simulink model "moto_linearization"  (R2026a)
settings: Solver=VariableStepAuto  StopTime=30
values from neighbouring files (symbols this model uses):
  ft = bs.FrontTire    [bikeSimToMotoParameters.m]
  Gf = Nsh.'*(Oh - B)    [bikeSimToMotoParameters.m]
  Ib = sum(I,3)    [bikeSimToMotoParameters.m]
  If = sum(I,3)    [bikeSimToMotoParameters.m]
  Ift = zeros(3)    [bikeSimToMotoParameters.m]
  Irt = zeros(3)    [bikeSimToMotoParameters.m]
  m = front_bodies(k).m    [bikeSimToMotoParameters.m]
  N = eye(3)    [bikeSimToMotoParameters.m]
  Ob = sum([rear_bodies.O].*[rear_bodies.m],2)/p.mb    [bikeSimToMotoParameters.m]
  p = motoParameters    [bikeSimToMotoParameters.m]    (also in moto_init.m = bikeSimToPrydeV2Parameters(bs,130/3.6); moto_trim_test.m = P{idx_vx}; steadyTurningTrimEqns.m = in3(41,:); steadyTurningTrimJac.m = in3(41,:))
  pf = fpacejka(bs.FrontTire.Pacejka)    [moto_trim_test.m]
  pr = fpacejka(bs.RearTire.Pacejka)    [moto_trim_test.m]
  rt = bs.RearTire    [bikeSimToMotoParameters.m]
  s = linspace(-pi,pi,36)'    [moto_init.m]
  sm = bs.SprungMass    [bikeSimToMotoParameters.m]
  X = zeros(ns,ns,12)    [moto_trim_test.m]
undefined symbols (not defined in the file or in its folder): mb, mh, Rr, Vlow, Y, Z
libraries: sm_lib x60, nesl_utility x51
(part 5 of 5)

== system moto_linearization/moto/Subsystem/front_tire/Subsystem1/Lateral force (pure slip)/Magic formula (lateral, camber) ==
  Bg : Inport
  Cg : Inport  Port=2
  Eg : Inport  Port=3
  camber : Inport  Port=4
  Atan : Trigonometry  Operator=atan
  Atan1 : Trigonometry  Operator=atan
  Product : Product
  Product1 : Product
  Product2 : Product
  Sum : Sum  Inputs=|+-
  Sum1 : Sum  Inputs=|+-
  Fy0g : Outport
  wires:
  Product2/1 -> Fy0g/1
  Eg/1 -> Product1/1
  Cg/1 -> Product2/1
  camber/1 -> Product/2
  Sum1/1 -> Atan1/1
  Product1/1 -> Sum1/2
  Sum/1 -> Product1/2
  Product/1 -> Sum1/1, Sum/1, Atan/1
  Atan1/1 -> Product2/2
  Atan/1 -> Sum/2
  Bg/1 -> Product/1

== system moto_linearization/moto/Subsystem/front_tire/Subsystem1/Lateral force (pure slip)/Magic formula (lateral, slip) ==
  By : Inport
  Cy : Inport  Port=2
  Ey : Inport  Port=3
  slip : Inport  Port=4
  Atan : Trigonometry  Operator=atan
  Atan1 : Trigonometry  Operator=atan
  Product : Product
  Product1 : Product
  Product2 : Product
  Sum : Sum  Inputs=|+-
  Sum1 : Sum  Inputs=|+-
  Fy0a : Outport
  wires:
  Product1/1 -> Sum1/2
  Sum1/1 -> Atan1/1
  slip/1 -> Product/2
  Atan/1 -> Sum/2
  Ey/1 -> Product1/1
  Atan1/1 -> Product2/2
  Product/1 -> Sum1/1, Sum/1, Atan/1
  Product2/1 -> Fy0a/1
  By/1 -> Product/1
  Sum/1 -> Product1/2
  Cy/1 -> Product2/1

== system moto_linearization/moto/Subsystem/front_tire/Subsystem1/Lateral force (pure slip)/lateral stiffness factor (camber, normalized) ==
  Kyg : Inport
  Cg : Inport  Port=2
  Dy : Inport  Port=3
  Divide : Product  Inputs=*/
  Product : Product
  Bg : Outport
  wires:
  Dy/1 -> Product/2
  Product/1 -> Divide/2
  Divide/1 -> Bg/1
  Cg/1 -> Product/1
  Kyg/1 -> Divide/1

== system moto_linearization/moto/Subsystem/front_tire/Subsystem1/Lateral force (pure slip)/lateral stiffness factor (slip, normalized) ==
  Kya : Inport
  Cy : Inport  Port=2
  Dy : Inport  Port=3
  Divide : Product  Inputs=*/
  Product : Product
  By : Outport
  wires:
  Cy/1 -> Product/1
  Dy/1 -> Product/2
  Kya/1 -> Divide/1
  Product/1 -> Divide/2
  Divide/1 -> By/1

== system moto_linearization/moto/Subsystem/front_tire/Subsystem1/Lateral force (pure slip, no camber)/Lateral curvature factor ==
  slip : Inport
  camber : Inport  Port=2
  pey1 : Inport  Port=3
  pey2 : Inport  Port=4
  pey4 : Inport  Port=5
  Product : Product  Inputs=3
  Product1 : Product
  Sign : Signum
  Square : Math  Operator=square
  Sum : Sum  Inputs=|++
  Sum1 : Sum  Inputs=|++
  Ey : Outport
  wires:
  slip/1 -> Sign/1
  pey1/1 -> Sum/1
  Sign/1 -> Product/1
  camber/1 -> Square/1, Product/3
  pey4/1 -> Product/2
  Product/1 -> Sum/2
  Sum/1 -> Sum1/1
  Square/1 -> Product1/1
  pey2/1 -> Product1/2
  Product1/1 -> Sum1/2
  Sum1/1 -> Ey/1

== system moto_linearization/moto/Subsystem/front_tire/Subsystem1/Lateral force (pure slip, no camber)/Lateral peak factor ==
  dfz : Inport
  Fz : Inport  Port=2
  camber : Inport  Port=3
  pdy1 : Inport  Port=4
  pdy2 : Inport  Port=5
  pdy3 : Inport  Port=6
  Constant : Constant
  Divide : Product  Inputs=*/
  Exp : Math
  Product : Product  Inputs=3
  Product1 : Product
  Product2 : Product
  Square : Math  Operator=square
  Sum : Sum  Inputs=|++
  Dy : Outport
  wires:
  Fz/1 -> Product/1
  pdy1/1 -> Product/2
  pdy2/1 -> Product1/1
  dfz/1 -> Product1/2
  Product1/1 -> Exp/1
  Exp/1 -> Product/3
  camber/1 -> Square/1
  pdy3/1 -> Product2/2
  Square/1 -> Product2/1
  Product/1 -> Divide/1
  Divide/1 -> Dy/1
  Product2/1 -> Sum/1
  Sum/1 -> Divide/2
  Constant/1 -> Sum/2

== system moto_linearization/moto/Subsystem/front_tire/Subsystem1/Lateral force (pure slip, no camber)/Lateral stiffness factor (camber) ==
  dfz : Inport
  Fz : Inport  Port=2
  pky6 : Inport  Port=3
  pky7 : Inport  Port=4
  Product : Product
  Product1 : Product
  Sum : Sum  Inputs=|++
  Kyg : Outport
  wires:
  pky7/1 -> Product/1
  dfz/1 -> Product/2
  Product/1 -> Sum/2
  pky6/1 -> Sum/1
  Sum/1 -> Product1/1
  Fz/1 -> Product1/2
  Product1/1 -> Kyg/1

== system moto_linearization/moto/Subsystem/front_tire/Subsystem1/Lateral force (pure slip, no camber)/Lateral stiffness factor (slip) ==
  Fz : Inport
  camber : Inport  Port=2
  Fz0 : Inport  Port=3
  pky1 : Inport  Port=4
  pky2 : Inport  Port=5
  pky3 : Inport  Port=6
  pky4 : Inport  Port=7
  pky5 : Inport  Port=8
  Atan : Trigonometry  Operator=atan
  Constant : Constant
  Divide : Product  Inputs=*/
  Divide1 : Product  Inputs=*/
  Product{,1..2,4} (4 alike) : Product
  Product3 : Product  Inputs=3
  Sin : Trigonometry
  Square : Math  Operator=square
  Sum : Sum  Inputs=|++
  Sum1 : Sum  Inputs=|++
  Kya : Outport
  wires:
  camber/1 -> Square/1
  Square/1 -> Product4/1, Product/2
  pky4/1 -> Product/1
  pky3/1 -> Sum/1
  Product/1 -> Sum/2
  Sum/1 -> Product1/2
  Fz0/1 -> Product3/2, Product1/1
  Product1/1 -> Divide/2
  Fz/1 -> Divide/1
  Divide/1 -> Atan/1
  Atan/1 -> Product2/2
  pky2/1 -> Product2/1
  Product2/1 -> Sin/1
  Sin/1 -> Product3/3
  pky1/1 -> Product3/1
  Product3/1 -> Divide1/1
  pky5/1 -> Product4/2
  Product4/1 -> Sum1/1
  Constant/1 -> Sum1/2
  Sum1/1 -> Divide1/2
  Divide1/1 -> Kya/1

== system moto_linearization/moto/Subsystem/front_tire/Subsystem1/Lateral force (pure slip, no camber)/Magic formula (lateral) ==
  Dy : Inport
  Fy0a : Inport  Port=2
  Fy0g : Inport  Port=3
  Product : Product
  Sin : Trigonometry
  Sum : Sum  Inputs=|++
  Fy0 : Outport
  wires:
  Fy0a/1 -> Sum/1
  Fy0g/1 -> Sum/2
  Sum/1 -> Sin/1
  Dy/1 -> Product/1
  Sin/1 -> Product/2
  Product/1 -> Fy0/1

== system moto_linearization/moto/Subsystem/front_tire/Subsystem1/Lateral force (pure slip, no camber)/Magic formula (lateral, camber) ==
  Bg : Inport
  Cg : Inport  Port=2
  Eg : Inport  Port=3
  camber : Inport  Port=4
  Atan : Trigonometry  Operator=atan
  Atan1 : Trigonometry  Operator=atan
  Product : Product
  Product1 : Product
  Product2 : Product
  Sum : Sum  Inputs=|+-
  Sum1 : Sum  Inputs=|+-
  Fy0g : Outport
  wires:
  Product2/1 -> Fy0g/1
  Eg/1 -> Product1/1
  Cg/1 -> Product2/1
  camber/1 -> Product/2
  Sum1/1 -> Atan1/1
  Product1/1 -> Sum1/2
  Sum/1 -> Product1/2
  Product/1 -> Sum1/1, Sum/1, Atan/1
  Atan1/1 -> Product2/2
  Atan/1 -> Sum/2
  Bg/1 -> Product/1

== system moto_linearization/moto/Subsystem/front_tire/Subsystem1/Lateral force (pure slip, no camber)/Magic formula (lateral, slip) ==
  By : Inport
  Cy : Inport  Port=2
  Ey : Inport  Port=3
  slip : Inport  Port=4
  Atan : Trigonometry  Operator=atan
  Atan1 : Trigonometry  Operator=atan
  Product : Product
  Product1 : Product
  Product2 : Product
  Sum : Sum  Inputs=|+-
  Sum1 : Sum  Inputs=|+-
  Fy0a : Outport
  wires:
  Product1/1 -> Sum1/2
  Sum1/1 -> Atan1/1
  slip/1 -> Product/2
  Atan/1 -> Sum/2
  Ey/1 -> Product1/1
  Atan1/1 -> Product2/2
  Product/1 -> Sum1/1, Sum/1, Atan/1
  Product2/1 -> Fy0a/1
  By/1 -> Product/1
  Sum/1 -> Product1/2
  Cy/1 -> Product2/1

== system moto_linearization/moto/Subsystem/front_tire/Subsystem1/Lateral force (pure slip, no camber)/lateral stiffness factor (camber, normalized) ==
  Kyg : Inport
  Cg : Inport  Port=2
  Dy : Inport  Port=3
  Divide : Product  Inputs=*/
  Product : Product
  Bg : Outport
  wires:
  Dy/1 -> Product/2
  Product/1 -> Divide/2
  Divide/1 -> Bg/1
  Cg/1 -> Product/1
  Kyg/1 -> Divide/1

== system moto_linearization/moto/Subsystem/front_tire/Subsystem1/Lateral force (pure slip, no camber)/lateral stiffness factor (slip, normalized) ==
  Kya : Inport
  Cy : Inport  Port=2
  Dy : Inport  Port=3
  Divide : Product  Inputs=*/
  Product : Product
  By : Outport
  wires:
  Cy/1 -> Product/1
  Dy/1 -> Product/2
  Kya/1 -> Divide/1
  Product/1 -> Divide/2
  Divide/1 -> By/1

== system moto_linearization/moto/Subsystem/front_tire/Subsystem1/Longitudinal force (combined slip)/Combined slip ==
  Bxa : Inport
  Cxa : Inport  Port=2
  Fx0 : Inport  Port=3
  slip_angle : Inport  Port=4
  Atan : Trigonometry  Operator=atan
  Cos : Trigonometry  Operator=cos
  Product : Product
  Product1 : Product
  Product2 : Product
  Fx : Outport
  wires:
  Bxa/1 -> Product/1
  slip_angle/1 -> Product/2
  Product/1 -> Atan/1
  Atan/1 -> Product1/1
  Cxa/1 -> Product1/2
  Product1/1 -> Cos/1
  Cos/1 -> Product2/1
  Fx0/1 -> Product2/2
  Product2/1 -> Fx/1

== system moto_linearization/moto/Subsystem/front_tire/Subsystem1/Longitudinal force (combined slip)/Longitudinal stiffness factor (combined) ==
  slip_ratio : Inport
  rbx1 : Inport  Port=2
  rbx2 : Inport  Port=3
  Atan : Trigonometry  Operator=atan
  Cos : Trigonometry  Operator=cos
  Product : Product
  Product1 : Product
  Bxa : Outport
  wires:
  slip_ratio/1 -> Product/1
  rbx2/1 -> Product/2
  Product/1 -> Atan/1
  Atan/1 -> Cos/1
  Cos/1 -> Product1/2
  rbx1/1 -> Product1/1
  Product1/1 -> Bxa/1

== system moto_linearization/moto/Subsystem/front_tire/Subsystem1/Longitudinal force (pure slip)/Longitudinal curvature factor ==
  dfz : Inport
  slip_ratio : Inport  Port=2
  pex1 : Inport  Port=3
  pex2 : Inport  Port=4
  pex3 : Inport  Port=5
  Constant : Constant
  Product : Product
  Product1 : Product
  Product2 : Product
  Sign : Signum
  Square : Math  Operator=square
  Sum : Sum  Inputs=|++
  Sum1 : Sum  Inputs=|++
  Sum2 : Sum  Inputs=|+-
  Ex : Outport
  wires:
  pex1/1 -> Sum/1
  Product/1 -> Sum/2
  pex2/1 -> Product/1
  dfz/1 -> Square/1, Product/2
  Square/1 -> Product1/1
  pex3/1 -> Product1/2
  Sum/1 -> Sum1/1
  Product1/1 -> Sum1/2
  Sum1/1 -> Product2/1
  Constant/1 -> Sum2/1
  Sum2/1 -> Product2/2
  Product2/1 -> Ex/1
  slip_ratio/1 -> Sign/1
  Sign/1 -> Sum2/2

== system moto_linearization/moto/Subsystem/front_tire/Subsystem1/Longitudinal force (pure slip)/Longitudinal peak factor ==
  dfz : Inport
  Fz : Inport  Port=2
  pdx1 : Inport  Port=3
  pdx2 : Inport  Port=4
  Product : Product
  Product1 : Product
  Sum : Sum  Inputs=|++
  Dx : Outport
  wires:
  dfz/1 -> Product/1
  pdx2/1 -> Product/2
  pdx1/1 -> Sum/1
  Product/1 -> Sum/2
  Fz/1 -> Product1/1
  Sum/1 -> Product1/2
  Product1/1 -> Dx/1

== system moto_linearization/moto/Subsystem/front_tire/Subsystem1/Longitudinal force (pure slip)/Longitudinal stiffness factor ==
  dfz : Inport
  Fz : Inport  Port=2
  pkx1 : Inport  Port=3
  pkx2 : Inport  Port=4
  pkx3 : Inport  Port=5
  Exp : Math
  Product : Product
  Product1 : Product
  Product2 : Product  Inputs=3
  Sum : Sum  Inputs=|++
  Kx : Outport
  wires:
  pkx2/1 -> Product/1
  dfz/1 -> Product1/1, Product/2
  pkx1/1 -> Sum/1
  Product/1 -> Sum/2
  pkx3/1 -> Product1/2
  Product1/1 -> Exp/1
  Fz/1 -> Product2/1
  Sum/1 -> Product2/2
  Exp/1 -> Product2/3
  Product2/1 -> Kx/1

== system moto_linearization/moto/Subsystem/front_tire/Subsystem1/Longitudinal force (pure slip)/Longitudinal stiffness factor (normalized) ==
  Kx : Inport
  Cx : Inport  Port=2
  Dx : Inport  Port=3
  Divide : Product  Inputs=*/
  Product : Product
  Bx : Outport
  wires:
  Cx/1 -> Product/1
  Dx/1 -> Product/2
  Kx/1 -> Divide/1
  Product/1 -> Divide/2
  Divide/1 -> Bx/1

== system moto_linearization/moto/Subsystem/front_tire/Subsystem1/Longitudinal force (pure slip)/Magic formula (longitudinal) ==
  Bx : Inport
  Cx : Inport  Port=2
  Dx : Inport  Port=3
  Ex : Inport  Port=4
  slip_ratio : Inport  Port=5
  Atan : Trigonometry  Operator=atan
  Atan1 : Trigonometry  Operator=atan
  Product{,1..3} (4 alike) : Product
  Sin : Trigonometry
  Sum : Sum  Inputs=|+-
  Sum1 : Sum  Inputs=|+-
  Fx0 : Outport
  wires:
  Bx/1 -> Product/1
  slip_ratio/1 -> Product/2
  Product/1 -> Sum1/1, Sum/1, Atan/1
  Atan/1 -> Sum/2
  Sum/1 -> Product1/2
  Ex/1 -> Product1/1
  Product1/1 -> Sum1/2
  Sum1/1 -> Atan1/1
  Atan1/1 -> Product2/2
  Cx/1 -> Product2/1
  Product2/1 -> Sin/1
  Sin/1 -> Product3/2
  Dx/1 -> Product3/1
  Product3/1 -> Fx0/1

== system moto_linearization/moto/Subsystem/rear_tire/Subsystem1/Aligning moment (combined slip)/Aligning moment (residual) ==
  Br : Inport
  Dr : Inport  Port=2
  residual_slip : Inport  Port=3
  Atan : Trigonometry  Operator=atan
  Cos : Trigonometry  Operator=cos
  Product : Product
  Product1 : Product
  Mzr : Outport
  wires:
  Br/1 -> Product/1
  residual_slip/1 -> Product/2
  Product/1 -> Atan/1
  Atan/1 -> Cos/1
  Cos/1 -> Product1/1
  Dr/1 -> Product1/2
  Product1/1 -> Mzr/1

== system moto_linearization/moto/Subsystem/rear_tire/Subsystem1/Aligning moment (combined slip)/Aligning moment (trail) ==
  Bt : Inport
  Ct : Inport  Port=2
  Dt : Inport  Port=3
  Et : Inport  Port=4
  slip_angle : Inport  Port=5
  trail_slip : Inport  Port=6
  Fyg0 : Inport  Port=7
  Atan : Trigonometry  Operator=atan
  Atan1 : Trigonometry  Operator=atan
  Constant : Constant
  Divide : Product  Inputs=*/
  Product{,1..4} (5 alike) : Product
  Sin : Trigonometry  Operator=cos
  Square : Math  Operator=square
  Square Root : Sqrt
  Sum : Sum  Inputs=|+-
  Sum1 : Sum  Inputs=|+-
  Sum2 : Sum  Inputs=|++
  Mzt : Outport
  wires:
  Dt/1 -> Product3/1
  Sum1/1 -> Atan1/1
  Bt/1 -> Product/1
  Product2/1 -> Sin/1
  Product3/1 -> Divide/1
  Product1/1 -> Sum1/2
  Et/1 -> Product1/1
  trail_slip/1 -> Product/2
  Ct/1 -> Product2/1
  Sum/1 -> Product1/2
  Product/1 -> Sum1/1, Sum/1, Atan/1
  Atan1/1 -> Product2/2
  Atan/1 -> Sum/2
  Sin/1 -> Product3/2
  slip_angle/1 -> Square/1
  Square/1 -> Sum2/1
  Constant/1 -> Sum2/2
  Sum2/1 -> Square Root/1
  Square Root/1 -> Divide/2
  Divide/1 -> Product4/1
  Fyg0/1 -> Product4/2
  Product4/1 -> Mzt/1

== system moto_linearization/moto/Subsystem/rear_tire/Subsystem1/Aligning moment (combined slip)/Curvature factor (trail) ==
  dfz : Inport
  slip : Inport  Port=2
  camber : Inport  Port=3
  Bt : Inport  Port=4
  Ct : Inport  Port=5
  qez1 : Inport  Port=6
  qez2 : Inport  Port=7
  qez5 : Inport  Port=8
  Atan : Trigonometry  Operator=atan
  Constant : Constant
  Gain : Gain  Gain=2/pi
  Product : Product  Inputs=3
  Product1 : Product  Inputs=3
  Product2 : Product
  Product3 : Product
  Sum : Sum  Inputs=|++
  Sum1 : Sum  Inputs=|++
  Et : Outport
  wires:
  Bt/1 -> Product/1
  Ct/1 -> Product/2
  slip/1 -> Product/3
  Product/1 -> Atan/1
  Atan/1 -> Gain/1
  Gain/1 -> Product1/1
  camber/1 -> Product1/2
  qez5/1 -> Product1/3
  Product1/1 -> Sum/1
  Constant/1 -> Sum/2
  Sum/1 -> Product2/1
  qez2/1 -> Product3/1
  dfz/1 -> Product3/2
  qez1/1 -> Sum1/1
  Product3/1 -> Sum1/2
  Sum1/1 -> Product2/2
  Product2/1 -> Et/1

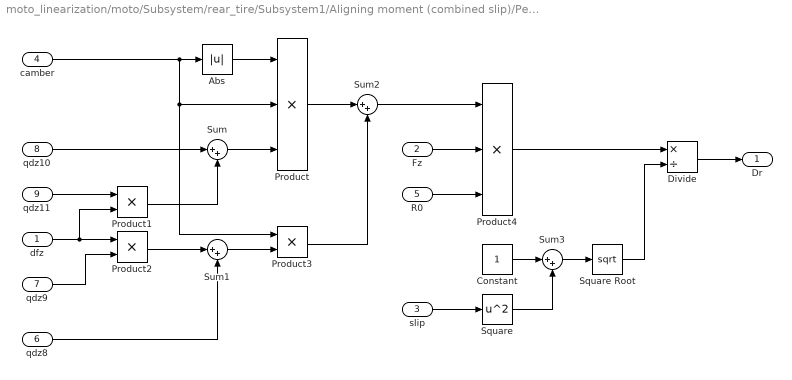
== system moto_linearization/moto/Subsystem/rear_tire/Subsystem1/Aligning moment (combined slip)/Peak factor (residual) ==
  dfz : Inport
  Fz : Inport  Port=2
  slip : Inport  Port=3
  camber : Inport  Port=4
  R0 : Inport  Port=5
  qdz8 : Inport  Port=6
  qdz9 : Inport  Port=7
  qdz10 : Inport  Port=8
  qdz11 : Inport  Port=9
  Abs : Abs  SaturateOnIntegerOverflow=off
  Constant : Constant
  Divide : Product  Inputs=*/
  Product : Product  Inputs=3
  Product1 : Product
  Product2 : Product
  Product3 : Product
  Product4 : Product  Inputs=3
  Square : Math  Operator=square
  Square Root : Sqrt
  Sum{,1..3} (4 alike) : Sum  Inputs=|++
  Dr : Outport
  wires:
  camber/1 -> Product3/1, Product/2, Abs/1
  Abs/1 -> Product/1
  qdz11/1 -> Product1/1
  dfz/1 -> Product2/1, Product1/2
  qdz10/1 -> Sum/1
  Product1/1 -> Sum/2
  Sum/1 -> Product/3
  qdz9/1 -> Product2/2
  Product2/1 -> Sum1/1
  qdz8/1 -> Sum1/2
  Sum1/1 -> Product3/2
  Product/1 -> Sum2/1
  Product3/1 -> Sum2/2
  Sum2/1 -> Product4/1
  Fz/1 -> Product4/2
  R0/1 -> Product4/3
  slip/1 -> Square/1
  Square/1 -> Sum3/2
  Constant/1 -> Sum3/1
  Sum3/1 -> Square Root/1
  Product4/1 -> Divide/1
  Square Root/1 -> Divide/2
  Divide/1 -> Dr/1

== system moto_linearization/moto/Subsystem/rear_tire/Subsystem1/Aligning moment (combined slip)/Peak factor (trail) ==
  dfz : Inport
  Fz : Inport  Port=2
  camber : Inport  Port=3
  R0 : Inport  Port=4
  Fz0 : Inport  Port=5
  qdz1 : Inport  Port=6
  qdz2 : Inport  Port=7
  qdz3 : Inport  Port=8
  qdz4 : Inport  Port=9
  Abs : Abs  SaturateOnIntegerOverflow=off
  Constant : Constant
  Divide : Product  Inputs=*/
  Product : Product  Inputs=4
  Product1 : Product
  Product2 : Product
  Product3 : Product
  Square : Math  Operator=square
  Sum : Sum  Inputs=|++
  Sum1 : Sum  Inputs=|++
  Sum2 : Sum  Inputs=|++
  Dt : Outport
  wires:
  R0/1 -> Divide/1
  Fz0/1 -> Divide/2
  Divide/1 -> Product/2
  Fz/1 -> Product/1
  dfz/1 -> Product1/2
  qdz2/1 -> Product1/1
  Sum/1 -> Product/3
  Product1/1 -> Sum/2
  qdz1/1 -> Sum/1
  camber/1 -> Square/1, Abs/1
  Abs/1 -> Product2/1
  qdz3/1 -> Product2/2
  Square/1 -> Product3/1
  qdz4/1 -> Product3/2
  Product2/1 -> Sum1/1
  Product3/1 -> Sum1/2
  Sum1/1 -> Sum2/1
  Constant/1 -> Sum2/2
  Sum2/1 -> Product/4
  Product/1 -> Dt/1

== system moto_linearization/moto/Subsystem/rear_tire/Subsystem1/Aligning moment (combined slip)/Stiffness factor (residual) ==
  By : Inport
  Cy : Inport  Port=2
  qbz9 : Inport  Port=3
  qbz10 : Inport  Port=4
  Product : Product  Inputs=3
  Sum : Sum  Inputs=|++
  Br : Outport
  wires:
  Cy/1 -> Product/2
  By/1 -> Product/3
  qbz10/1 -> Product/1
  qbz9/1 -> Sum/1
  Product/1 -> Sum/2
  Sum/1 -> Br/1

== system moto_linearization/moto/Subsystem/rear_tire/Subsystem1/Aligning moment (combined slip)/Stiffness factor (trail) ==
  dfz : Inport
  camber : Inport  Port=2
  qbz1 : Inport  Port=3
  qbz2 : Inport  Port=4
  qbz5 : Inport  Port=5
  qbz6 : Inport  Port=6
  Abs : Abs  SaturateOnIntegerOverflow=off
  Constant : Constant
  Product{,1..3} (4 alike) : Product
  Square : Math  Operator=square
  Sum : Sum  Inputs=|++
  Sum1 : Sum  Inputs=|++
  Sum2 : Sum  Inputs=|++
  Bt : Outport
  wires:
  qbz2/1 -> Product/1
  dfz/1 -> Product/2
  qbz1/1 -> Sum/1
  Product/1 -> Sum/2
  camber/1 -> Square/1, Abs/1
  Abs/1 -> Product1/1
  qbz5/1 -> Product1/2
  qbz6/1 -> Product2/1
  Square/1 -> Product2/2
  Constant/1 -> Sum1/1
  Product2/1 -> Sum1/2
  Sum1/1 -> Sum2/1
  Product1/1 -> Sum2/2
  Sum2/1 -> Product3/1
  Sum/1 -> Product3/2
  Product3/1 -> Bt/1

== system moto_linearization/moto/Subsystem/rear_tire/Subsystem1/Lateral force (combined slip)/Combined slip ==
  Byk : Inport
  Fy0 : Inport  Port=2
  slip_ratio : Inport  Port=3
  Cyk : Inport  Port=4
  Atan : Trigonometry  Operator=atan
  Cos : Trigonometry  Operator=cos
  Product : Product
  Product1 : Product
  Product2 : Product
  Fy : Outport
  wires:
  Byk/1 -> Product/1
  slip_ratio/1 -> Product/2
  Product/1 -> Atan/1
  Atan/1 -> Product1/1
  Cyk/1 -> Product1/2
  Product1/1 -> Cos/1
  Cos/1 -> Product2/1
  Fy0/1 -> Product2/2
  Product2/1 -> Fy/1

== system moto_linearization/moto/Subsystem/rear_tire/Subsystem1/Lateral force (combined slip)/Lateral stiffness factor (combined) ==
  slip_angle : Inport
  rby1 : Inport  Port=2
  rby2 : Inport  Port=3
  rby3 : Inport  Port=4
  Atan : Trigonometry  Operator=atan
  Cos : Trigonometry  Operator=cos
  Product : Product
  Product1 : Product
  Sum : Sum  Inputs=|+-
  Byk : Outport
  wires:
  slip_angle/1 -> Sum/1
  rby3/1 -> Sum/2
  Sum/1 -> Product/2
  rby2/1 -> Product/1
  Product/1 -> Atan/1
  Atan/1 -> Cos/1
  Cos/1 -> Product1/2
  rby1/1 -> Product1/1
  Product1/1 -> Byk/1

== system moto_linearization/moto/Subsystem/rear_tire/Subsystem1/Lateral force (combined slip, no camber)/Combined slip ==
  Byk : Inport
  Fy0 : Inport  Port=2
  slip_ratio : Inport  Port=3
  Cyk : Inport  Port=4
  Atan : Trigonometry  Operator=atan
  Cos : Trigonometry  Operator=cos
  Product : Product
  Product1 : Product
  Product2 : Product
  Fy : Outport
  wires:
  Byk/1 -> Product/1
  slip_ratio/1 -> Product/2
  Product/1 -> Atan/1
  Atan/1 -> Product1/1
  Cyk/1 -> Product1/2
  Product1/1 -> Cos/1
  Cos/1 -> Product2/1
  Fy0/1 -> Product2/2
  Product2/1 -> Fy/1

== system moto_linearization/moto/Subsystem/rear_tire/Subsystem1/Lateral force (combined slip, no camber)/Lateral stiffness factor (combined) ==
  slip_angle : Inport
  rby1 : Inport  Port=2
  rby2 : Inport  Port=3
  rby3 : Inport  Port=4
  Atan : Trigonometry  Operator=atan
  Cos : Trigonometry  Operator=cos
  Product : Product
  Product1 : Product
  Sum : Sum  Inputs=|+-
  Byk : Outport
  wires:
  slip_angle/1 -> Sum/1
  rby3/1 -> Sum/2
  Sum/1 -> Product/2
  rby2/1 -> Product/1
  Product/1 -> Atan/1
  Atan/1 -> Cos/1
  Cos/1 -> Product1/2
  rby1/1 -> Product1/1
  Product1/1 -> Byk/1

== system moto_linearization/moto/Subsystem/rear_tire/Subsystem1/Lateral force (pure slip)/Lateral curvature factor ==
  slip : Inport
  camber : Inport  Port=2
  pey1 : Inport  Port=3
  pey2 : Inport  Port=4
  pey4 : Inport  Port=5
  Product : Product  Inputs=3
  Product1 : Product
  Sign : Signum
  Square : Math  Operator=square
  Sum : Sum  Inputs=|++
  Sum1 : Sum  Inputs=|++
  Ey : Outport
  wires:
  slip/1 -> Sign/1
  pey1/1 -> Sum/1
  Sign/1 -> Product/1
  camber/1 -> Square/1, Product/3
  pey4/1 -> Product/2
  Product/1 -> Sum/2
  Sum/1 -> Sum1/1
  Square/1 -> Product1/1
  pey2/1 -> Product1/2
  Product1/1 -> Sum1/2
  Sum1/1 -> Ey/1

== system moto_linearization/moto/Subsystem/rear_tire/Subsystem1/Lateral force (pure slip)/Lateral peak factor ==
  dfz : Inport
  Fz : Inport  Port=2
  camber : Inport  Port=3
  pdy1 : Inport  Port=4
  pdy2 : Inport  Port=5
  pdy3 : Inport  Port=6
  Constant : Constant
  Divide : Product  Inputs=*/
  Exp : Math
  Product : Product  Inputs=3
  Product1 : Product
  Product2 : Product
  Square : Math  Operator=square
  Sum : Sum  Inputs=|++
  Dy : Outport
  wires:
  Fz/1 -> Product/1
  pdy1/1 -> Product/2
  pdy2/1 -> Product1/1
  dfz/1 -> Product1/2
  Product1/1 -> Exp/1
  Exp/1 -> Product/3
  camber/1 -> Square/1
  pdy3/1 -> Product2/2
  Square/1 -> Product2/1
  Product/1 -> Divide/1
  Divide/1 -> Dy/1
  Product2/1 -> Sum/1
  Sum/1 -> Divide/2
  Constant/1 -> Sum/2

== system moto_linearization/moto/Subsystem/rear_tire/Subsystem1/Lateral force (pure slip)/Lateral stiffness factor (camber) ==
  dfz : Inport
  Fz : Inport  Port=2
  pky6 : Inport  Port=3
  pky7 : Inport  Port=4
  Product : Product
  Product1 : Product
  Sum : Sum  Inputs=|++
  Kyg : Outport
  wires:
  pky7/1 -> Product/1
  dfz/1 -> Product/2
  Product/1 -> Sum/2
  pky6/1 -> Sum/1
  Sum/1 -> Product1/1
  Fz/1 -> Product1/2
  Product1/1 -> Kyg/1

== system moto_linearization/moto/Subsystem/rear_tire/Subsystem1/Lateral force (pure slip)/Lateral stiffness factor (slip) ==
  Fz : Inport
  camber : Inport  Port=2
  Fz0 : Inport  Port=3
  pky1 : Inport  Port=4
  pky2 : Inport  Port=5
  pky3 : Inport  Port=6
  pky4 : Inport  Port=7
  pky5 : Inport  Port=8
  Atan : Trigonometry  Operator=atan
  Constant : Constant
  Divide : Product  Inputs=*/
  Divide1 : Product  Inputs=*/
  Product{,1..2,4} (4 alike) : Product
  Product3 : Product  Inputs=3
  Sin : Trigonometry
  Square : Math  Operator=square
  Sum : Sum  Inputs=|++
  Sum1 : Sum  Inputs=|++
  Kya : Outport
  wires:
  camber/1 -> Square/1
  Square/1 -> Product4/1, Product/2
  pky4/1 -> Product/1
  pky3/1 -> Sum/1
  Product/1 -> Sum/2
  Sum/1 -> Product1/2
  Fz0/1 -> Product3/2, Product1/1
  Product1/1 -> Divide/2
  Fz/1 -> Divide/1
  Divide/1 -> Atan/1
  Atan/1 -> Product2/2
  pky2/1 -> Product2/1
  Product2/1 -> Sin/1
  Sin/1 -> Product3/3
  pky1/1 -> Product3/1
  Product3/1 -> Divide1/1
  pky5/1 -> Product4/2
  Product4/1 -> Sum1/1
  Constant/1 -> Sum1/2
  Sum1/1 -> Divide1/2
  Divide1/1 -> Kya/1

== system moto_linearization/moto/Subsystem/rear_tire/Subsystem1/Lateral force (pure slip)/Magic formula (lateral) ==
  Dy : Inport
  Fy0a : Inport  Port=2
  Fy0g : Inport  Port=3
  Product : Product
  Sin : Trigonometry
  Sum : Sum  Inputs=|++
  Fy0 : Outport
  wires:
  Fy0a/1 -> Sum/1
  Fy0g/1 -> Sum/2
  Sum/1 -> Sin/1
  Dy/1 -> Product/1
  Sin/1 -> Product/2
  Product/1 -> Fy0/1

== system moto_linearization/moto/Subsystem/rear_tire/Subsystem1/Lateral force (pure slip)/Magic formula (lateral, camber) ==
  Bg : Inport
  Cg : Inport  Port=2
  Eg : Inport  Port=3
  camber : Inport  Port=4
  Atan : Trigonometry  Operator=atan
  Atan1 : Trigonometry  Operator=atan
  Product : Product
  Product1 : Product
  Product2 : Product
  Sum : Sum  Inputs=|+-
  Sum1 : Sum  Inputs=|+-
  Fy0g : Outport
  wires:
  Product2/1 -> Fy0g/1
  Eg/1 -> Product1/1
  Cg/1 -> Product2/1
  camber/1 -> Product/2
  Sum1/1 -> Atan1/1
  Product1/1 -> Sum1/2
  Sum/1 -> Product1/2
  Product/1 -> Sum1/1, Sum/1, Atan/1
  Atan1/1 -> Product2/2
  Atan/1 -> Sum/2
  Bg/1 -> Product/1

== system moto_linearization/moto/Subsystem/rear_tire/Subsystem1/Lateral force (pure slip)/Magic formula (lateral, slip) ==
  By : Inport
  Cy : Inport  Port=2
  Ey : Inport  Port=3
  slip : Inport  Port=4
  Atan : Trigonometry  Operator=atan
  Atan1 : Trigonometry  Operator=atan
  Product : Product
  Product1 : Product
  Product2 : Product
  Sum : Sum  Inputs=|+-
  Sum1 : Sum  Inputs=|+-
  Fy0a : Outport
  wires:
  Product1/1 -> Sum1/2
  Sum1/1 -> Atan1/1
  slip/1 -> Product/2
  Atan/1 -> Sum/2
  Ey/1 -> Product1/1
  Atan1/1 -> Product2/2
  Product/1 -> Sum1/1, Sum/1, Atan/1
  Product2/1 -> Fy0a/1
  By/1 -> Product/1
  Sum/1 -> Product1/2
  Cy/1 -> Product2/1

== system moto_linearization/moto/Subsystem/rear_tire/Subsystem1/Lateral force (pure slip)/lateral stiffness factor (camber, normalized) ==
  Kyg : Inport
  Cg : Inport  Port=2
  Dy : Inport  Port=3
  Divide : Product  Inputs=*/
  Product : Product
  Bg : Outport
  wires:
  Dy/1 -> Product/2
  Product/1 -> Divide/2
  Divide/1 -> Bg/1
  Cg/1 -> Product/1
  Kyg/1 -> Divide/1

== system moto_linearization/moto/Subsystem/rear_tire/Subsystem1/Lateral force (pure slip)/lateral stiffness factor (slip, normalized) ==
  Kya : Inport
  Cy : Inport  Port=2
  Dy : Inport  Port=3
  Divide : Product  Inputs=*/
  Product : Product
  By : Outport
  wires:
  Cy/1 -> Product/1
  Dy/1 -> Product/2
  Kya/1 -> Divide/1
  Product/1 -> Divide/2
  Divide/1 -> By/1

== system moto_linearization/moto/Subsystem/rear_tire/Subsystem1/Lateral force (pure slip, no camber)/Lateral curvature factor ==
  slip : Inport
  camber : Inport  Port=2
  pey1 : Inport  Port=3
  pey2 : Inport  Port=4
  pey4 : Inport  Port=5
  Product : Product  Inputs=3
  Product1 : Product
  Sign : Signum
  Square : Math  Operator=square
  Sum : Sum  Inputs=|++
  Sum1 : Sum  Inputs=|++
  Ey : Outport
  wires:
  slip/1 -> Sign/1
  pey1/1 -> Sum/1
  Sign/1 -> Product/1
  camber/1 -> Square/1, Product/3
  pey4/1 -> Product/2
  Product/1 -> Sum/2
  Sum/1 -> Sum1/1
  Square/1 -> Product1/1
  pey2/1 -> Product1/2
  Product1/1 -> Sum1/2
  Sum1/1 -> Ey/1

== system moto_linearization/moto/Subsystem/rear_tire/Subsystem1/Lateral force (pure slip, no camber)/Lateral peak factor ==
  dfz : Inport
  Fz : Inport  Port=2
  camber : Inport  Port=3
  pdy1 : Inport  Port=4
  pdy2 : Inport  Port=5
  pdy3 : Inport  Port=6
  Constant : Constant
  Divide : Product  Inputs=*/
  Exp : Math
  Product : Product  Inputs=3
  Product1 : Product
  Product2 : Product
  Square : Math  Operator=square
  Sum : Sum  Inputs=|++
  Dy : Outport
  wires:
  Fz/1 -> Product/1
  pdy1/1 -> Product/2
  pdy2/1 -> Product1/1
  dfz/1 -> Product1/2
  Product1/1 -> Exp/1
  Exp/1 -> Product/3
  camber/1 -> Square/1
  pdy3/1 -> Product2/2
  Square/1 -> Product2/1
  Product/1 -> Divide/1
  Divide/1 -> Dy/1
  Product2/1 -> Sum/1
  Sum/1 -> Divide/2
  Constant/1 -> Sum/2

== system moto_linearization/moto/Subsystem/rear_tire/Subsystem1/Lateral force (pure slip, no camber)/Lateral stiffness factor (camber) ==
  dfz : Inport
  Fz : Inport  Port=2
  pky6 : Inport  Port=3
  pky7 : Inport  Port=4
  Product : Product
  Product1 : Product
  Sum : Sum  Inputs=|++
  Kyg : Outport
  wires:
  pky7/1 -> Product/1
  dfz/1 -> Product/2
  Product/1 -> Sum/2
  pky6/1 -> Sum/1
  Sum/1 -> Product1/1
  Fz/1 -> Product1/2
  Product1/1 -> Kyg/1

== system moto_linearization/moto/Subsystem/rear_tire/Subsystem1/Lateral force (pure slip, no camber)/Lateral stiffness factor (slip) ==
  Fz : Inport
  camber : Inport  Port=2
  Fz0 : Inport  Port=3
  pky1 : Inport  Port=4
  pky2 : Inport  Port=5
  pky3 : Inport  Port=6
  pky4 : Inport  Port=7
  pky5 : Inport  Port=8
  Atan : Trigonometry  Operator=atan
  Constant : Constant
  Divide : Product  Inputs=*/
  Divide1 : Product  Inputs=*/
  Product{,1..2,4} (4 alike) : Product
  Product3 : Product  Inputs=3
  Sin : Trigonometry
  Square : Math  Operator=square
  Sum : Sum  Inputs=|++
  Sum1 : Sum  Inputs=|++
  Kya : Outport
  wires:
  camber/1 -> Square/1
  Square/1 -> Product4/1, Product/2
  pky4/1 -> Product/1
  pky3/1 -> Sum/1
  Product/1 -> Sum/2
  Sum/1 -> Product1/2
  Fz0/1 -> Product3/2, Product1/1
  Product1/1 -> Divide/2
  Fz/1 -> Divide/1
  Divide/1 -> Atan/1
  Atan/1 -> Product2/2
  pky2/1 -> Product2/1
  Product2/1 -> Sin/1
  Sin/1 -> Product3/3
  pky1/1 -> Product3/1
  Product3/1 -> Divide1/1
  pky5/1 -> Product4/2
  Product4/1 -> Sum1/1
  Constant/1 -> Sum1/2
  Sum1/1 -> Divide1/2
  Divide1/1 -> Kya/1

== system moto_linearization/moto/Subsystem/rear_tire/Subsystem1/Lateral force (pure slip, no camber)/Magic formula (lateral) ==
  Dy : Inport
  Fy0a : Inport  Port=2
  Fy0g : Inport  Port=3
  Product : Product
  Sin : Trigonometry
  Sum : Sum  Inputs=|++
  Fy0 : Outport
  wires:
  Fy0a/1 -> Sum/1
  Fy0g/1 -> Sum/2
  Sum/1 -> Sin/1
  Dy/1 -> Product/1
  Sin/1 -> Product/2
  Product/1 -> Fy0/1

== system moto_linearization/moto/Subsystem/rear_tire/Subsystem1/Lateral force (pure slip, no camber)/Magic formula (lateral, camber) ==
  Bg : Inport
  Cg : Inport  Port=2
  Eg : Inport  Port=3
  camber : Inport  Port=4
  Atan : Trigonometry  Operator=atan
  Atan1 : Trigonometry  Operator=atan
  Product : Product
  Product1 : Product
  Product2 : Product
  Sum : Sum  Inputs=|+-
  Sum1 : Sum  Inputs=|+-
  Fy0g : Outport
  wires:
  Product2/1 -> Fy0g/1
  Eg/1 -> Product1/1
  Cg/1 -> Product2/1
  camber/1 -> Product/2
  Sum1/1 -> Atan1/1
  Product1/1 -> Sum1/2
  Sum/1 -> Product1/2
  Product/1 -> Sum1/1, Sum/1, Atan/1
  Atan1/1 -> Product2/2
  Atan/1 -> Sum/2
  Bg/1 -> Product/1

== system moto_linearization/moto/Subsystem/rear_tire/Subsystem1/Lateral force (pure slip, no camber)/Magic formula (lateral, slip) ==
  By : Inport
  Cy : Inport  Port=2
  Ey : Inport  Port=3
  slip : Inport  Port=4
  Atan : Trigonometry  Operator=atan
  Atan1 : Trigonometry  Operator=atan
  Product : Product
  Product1 : Product
  Product2 : Product
  Sum : Sum  Inputs=|+-
  Sum1 : Sum  Inputs=|+-
  Fy0a : Outport
  wires:
  Product1/1 -> Sum1/2
  Sum1/1 -> Atan1/1
  slip/1 -> Product/2
  Atan/1 -> Sum/2
  Ey/1 -> Product1/1
  Atan1/1 -> Product2/2
  Product/1 -> Sum1/1, Sum/1, Atan/1
  Product2/1 -> Fy0a/1
  By/1 -> Product/1
  Sum/1 -> Product1/2
  Cy/1 -> Product2/1

== system moto_linearization/moto/Subsystem/rear_tire/Subsystem1/Lateral force (pure slip, no camber)/lateral stiffness factor (camber, normalized) ==
  Kyg : Inport
  Cg : Inport  Port=2
  Dy : Inport  Port=3
  Divide : Product  Inputs=*/
  Product : Product
  Bg : Outport
  wires:
  Dy/1 -> Product/2
  Product/1 -> Divide/2
  Divide/1 -> Bg/1
  Cg/1 -> Product/1
  Kyg/1 -> Divide/1

== system moto_linearization/moto/Subsystem/rear_tire/Subsystem1/Lateral force (pure slip, no camber)/lateral stiffness factor (slip, normalized) ==
  Kya : Inport
  Cy : Inport  Port=2
  Dy : Inport  Port=3
  Divide : Product  Inputs=*/
  Product : Product
  By : Outport
  wires:
  Cy/1 -> Product/1
  Dy/1 -> Product/2
  Kya/1 -> Divide/1
  Product/1 -> Divide/2
  Divide/1 -> By/1

== system moto_linearization/moto/Subsystem/rear_tire/Subsystem1/Longitudinal force (combined slip)/Combined slip ==
  Bxa : Inport
  Cxa : Inport  Port=2
  Fx0 : Inport  Port=3
  slip_angle : Inport  Port=4
  Atan : Trigonometry  Operator=atan
  Cos : Trigonometry  Operator=cos
  Product : Product
  Product1 : Product
  Product2 : Product
  Fx : Outport
  wires:
  Bxa/1 -> Product/1
  slip_angle/1 -> Product/2
  Product/1 -> Atan/1
  Atan/1 -> Product1/1
  Cxa/1 -> Product1/2
  Product1/1 -> Cos/1
  Cos/1 -> Product2/1
  Fx0/1 -> Product2/2
  Product2/1 -> Fx/1

== system moto_linearization/moto/Subsystem/rear_tire/Subsystem1/Longitudinal force (combined slip)/Longitudinal stiffness factor (combined) ==
  slip_ratio : Inport
  rbx1 : Inport  Port=2
  rbx2 : Inport  Port=3
  Atan : Trigonometry  Operator=atan
  Cos : Trigonometry  Operator=cos
  Product : Product
  Product1 : Product
  Bxa : Outport
  wires:
  slip_ratio/1 -> Product/1
  rbx2/1 -> Product/2
  Product/1 -> Atan/1
  Atan/1 -> Cos/1
  Cos/1 -> Product1/2
  rbx1/1 -> Product1/1
  Product1/1 -> Bxa/1

== system moto_linearization/moto/Subsystem/rear_tire/Subsystem1/Longitudinal force (pure slip)/Longitudinal curvature factor ==
  dfz : Inport
  slip_ratio : Inport  Port=2
  pex1 : Inport  Port=3
  pex2 : Inport  Port=4
  pex3 : Inport  Port=5
  Constant : Constant
  Product : Product
  Product1 : Product
  Product2 : Product
  Sign : Signum
  Square : Math  Operator=square
  Sum : Sum  Inputs=|++
  Sum1 : Sum  Inputs=|++
  Sum2 : Sum  Inputs=|+-
  Ex : Outport
  wires:
  pex1/1 -> Sum/1
  Product/1 -> Sum/2
  pex2/1 -> Product/1
  dfz/1 -> Square/1, Product/2
  Square/1 -> Product1/1
  pex3/1 -> Product1/2
  Sum/1 -> Sum1/1
  Product1/1 -> Sum1/2
  Sum1/1 -> Product2/1
  Constant/1 -> Sum2/1
  Sum2/1 -> Product2/2
  Product2/1 -> Ex/1
  slip_ratio/1 -> Sign/1
  Sign/1 -> Sum2/2

== system moto_linearization/moto/Subsystem/rear_tire/Subsystem1/Longitudinal force (pure slip)/Longitudinal peak factor ==
  dfz : Inport
  Fz : Inport  Port=2
  pdx1 : Inport  Port=3
  pdx2 : Inport  Port=4
  Product : Product
  Product1 : Product
  Sum : Sum  Inputs=|++
  Dx : Outport
  wires:
  dfz/1 -> Product/1
  pdx2/1 -> Product/2
  pdx1/1 -> Sum/1
  Product/1 -> Sum/2
  Fz/1 -> Product1/1
  Sum/1 -> Product1/2
  Product1/1 -> Dx/1

== system moto_linearization/moto/Subsystem/rear_tire/Subsystem1/Longitudinal force (pure slip)/Longitudinal stiffness factor ==
  dfz : Inport
  Fz : Inport  Port=2
  pkx1 : Inport  Port=3
  pkx2 : Inport  Port=4
  pkx3 : Inport  Port=5
  Exp : Math
  Product : Product
  Product1 : Product
  Product2 : Product  Inputs=3
  Sum : Sum  Inputs=|++
  Kx : Outport
  wires:
  pkx2/1 -> Product/1
  dfz/1 -> Product1/1, Product/2
  pkx1/1 -> Sum/1
  Product/1 -> Sum/2
  pkx3/1 -> Product1/2
  Product1/1 -> Exp/1
  Fz/1 -> Product2/1
  Sum/1 -> Product2/2
  Exp/1 -> Product2/3
  Product2/1 -> Kx/1

== system moto_linearization/moto/Subsystem/rear_tire/Subsystem1/Longitudinal force (pure slip)/Longitudinal stiffness factor (normalized) ==
  Kx : Inport
  Cx : Inport  Port=2
  Dx : Inport  Port=3
  Divide : Product  Inputs=*/
  Product : Product
  Bx : Outport
  wires:
  Cx/1 -> Product/1
  Dx/1 -> Product/2
  Kx/1 -> Divide/1
  Product/1 -> Divide/2
  Divide/1 -> Bx/1

== system moto_linearization/moto/Subsystem/rear_tire/Subsystem1/Longitudinal force (pure slip)/Magic formula (longitudinal) ==
  Bx : Inport
  Cx : Inport  Port=2
  Dx : Inport  Port=3
  Ex : Inport  Port=4
  slip_ratio : Inport  Port=5
  Atan : Trigonometry  Operator=atan
  Atan1 : Trigonometry  Operator=atan
  Product{,1..3} (4 alike) : Product
  Sin : Trigonometry
  Sum : Sum  Inputs=|+-
  Sum1 : Sum  Inputs=|+-
  Fx0 : Outport
  wires:
  Bx/1 -> Product/1
  slip_ratio/1 -> Product/2
  Product/1 -> Sum1/1, Sum/1, Atan/1
  Atan/1 -> Sum/2
  Sum/1 -> Product1/2
  Ex/1 -> Product1/1
  Product1/1 -> Sum1/2
  Sum1/1 -> Atan1/1
  Atan1/1 -> Product2/2
  Cx/1 -> Product2/1
  Product2/1 -> Sin/1
  Sin/1 -> Product3/2
  Dx/1 -> Product3/1
  Product3/1 -> Fx0/1
